simulink model "Heating_Seperated"  (R2017b)
settings: Solver=FixedStepDiscrete  StartTime=0.0  StopTime=50000  FixedStep=0.5  RelTol=1e-3
libraries: cstblocks x2
settings Model: Creator=arbno  LastModifiedBy=arbno

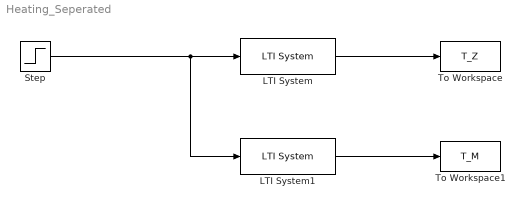
== system Heating_Seperated ==
  LTI System : cstblocks/LTI System  sys=G_Z_Zelle  IC=[]
  LTI System1 : cstblocks/LTI System  sys=G_Z_Mantel  IC=[]
  Step : Step  Time=0  After=0.005  SampleTime=0
  To Workspace : ToWorkspace  VariableName=T_Z  SaveFormat=Structure With Time  SampleTime=-1
  To Workspace1 : ToWorkspace  VariableName=T_M  SaveFormat=Structure With Time  SampleTime=-1
  wires:
  Step/1 -> LTI System/1, LTI System1/1
  LTI System/1 -> To Workspace/1
  LTI System1/1 -> To Workspace1/1
